simulink model "float_mch_Sample_AdaptiveThreshold"  (R2020a)
settings: Solver=VariableStepAuto  StartTime=0  StopTime=5  RelTol=1e-3
values from neighbouring files (symbols this model uses):
  fs = 30000    [float_mch_run_LocalMaxima_AdaptiveThreshold.m]    (also in float_mch_run_LocalMaxima_HardThreshold.m; float_mch_run_Sample_AdaptiveThreshold.m; float_mch_run_Sample_HardThreshold.m)
libraries: dspfdesign x2, dspswit3 x1, dspstat3 x1, simulink x1
settings Model: Creator=sbuccelli  LastModifiedBy=diflo

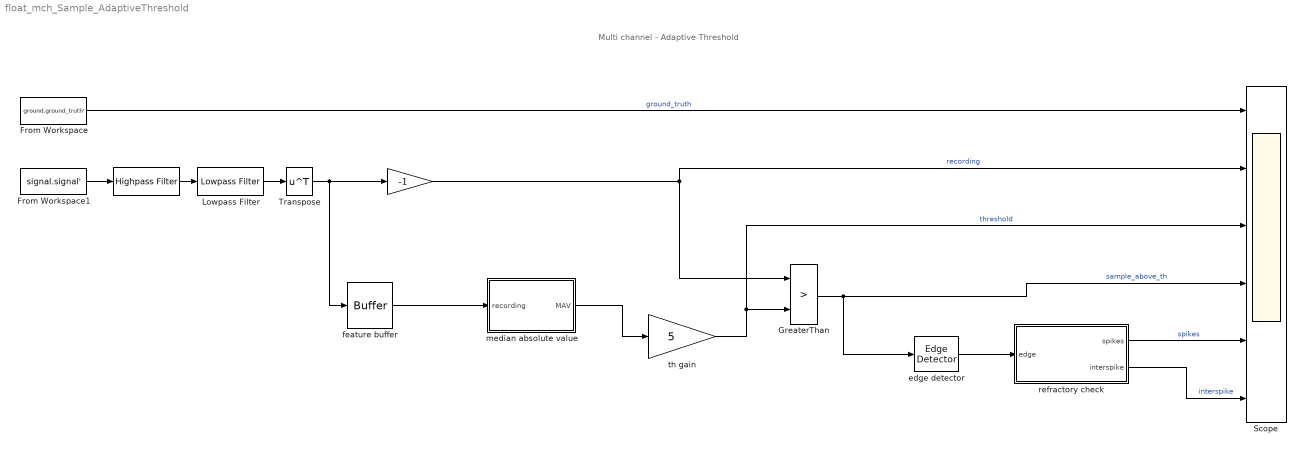
== system float_mch_Sample_AdaptiveThreshold ==
  note: Multi channel - Adaptive Threshold
  " " : Gain  Gain=-1
  "   " : dspfdesign/Highpass Filter  FilterType=IIR  DesignForMinimumOrder=on  FilterOrder=50  StopbandFrequency=1  PassbandFrequency=300  StopbandAttenuation=80  PassbandRipple=0.1  InheritSampleRate=off  SampleRate=30000  SimulateUsing=Interpreted execution  roundingMode=Floor  coeffsDataTypeStr=fixdt(1,16)
  From Workspace : FromWorkspace  VariableName=ground.ground_truth'  SampleTime=1/fs
  From Workspace1 : FromWorkspace  VariableName=signal.signal'  SampleTime=1/fs
  GreaterThan : RelationalOperator  Operator=>  OutDataTypeStr=boolean  RndMeth=Simplest
  Lowpass Filter : dspfdesign/Lowpass Filter  FilterType=IIR  DesignForMinimumOrder=on  FilterOrder=3  PassbandFrequency=3500  StopbandFrequency=8500  PassbandRipple=0.1  StopbandAttenuation=80  InheritSampleRate=off  SampleRate=30000  SimulateUsing=Interpreted execution  roundingMode=Floor  coeffsDataTypeStr=fixdt(1,16)
  Scope : Scope  NumInputPorts=6
  Transpose : Math  Operator=transpose  SaturateOnIntegerOverflow=on
  edge detector : dspswit3/Edge Detector  InputProcessing=Columns as channels (frame based)
      settings: SourceProductBaseCode=DS
  feature buffer : Buffer  N=30000  OutputFrames=off
  median absolute value : Subsystem
  refractory check : Subsystem
  th gain : Gain  Gain=5
  wires:
  From Workspace/1 -> Scope/1  "ground_truth"
  edge detector/1 -> refractory check/1("edge  ")
  refractory check/2(interspike) -> Scope/6  "interspike"
  GreaterThan/1 -> Scope/4, edge detector/1  "sample_above_th"
  th gain/1 -> GreaterThan/2, Scope/3  "threshold"
  refractory check/1(spikes) -> Scope/5  "spikes"
  From Workspace1/1 -> "   "/1
  " "/1 -> GreaterThan/1, Scope/2  "recording"
  feature buffer/1 -> median absolute value/1(recording)
  median absolute value/1(MAV) -> th gain/1
  Transpose/1 -> feature buffer/1, " "/1
  "   "/1 -> Lowpass Filter/1
  Lowpass Filter/1 -> Transpose/1

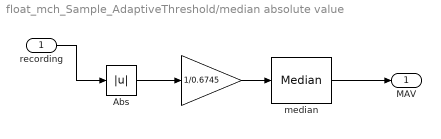
== system float_mch_Sample_AdaptiveThreshold/median absolute value ==
  recording : Inport
  "  " : Gain  Gain=1/0.6745
  Abs : Abs
  median : dspstat3/Median  sortAlg=Quick sort  directionMode=Each column  dimension=1  roundingMode=Floor  overflowMode=off  accumDataTypeStr=Inherit: Same as product output  accumLastDataTypeStr=Inherit: Same as product output  outputDataTypeStr=Inherit: Same as accumulator  outputMin=[]  outputMax=[]  outputLastDataTypeStr=Inherit: Same as accumulator
      settings: SourceProductBaseCode=DS  allowOverrides=off
  MAV : Outport
  wires:
  Abs/1 -> "  "/1
  "  "/1 -> median/1
  recording/1 -> Abs/1
  median/1 -> MAV/1

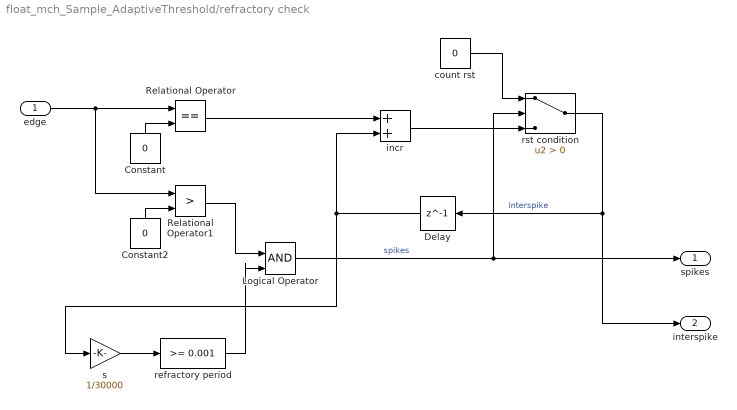
== system float_mch_Sample_AdaptiveThreshold/refractory check ==
  "edge  " : Inport
  Constant : Constant  Value=0
  Constant2 : Constant  Value=0
  Delay : Delay  DelayLength=1  InitialCondition=1
  Logical Operator : Logic  IconShape=distinctive  AllPortsSameDT=off  OutDataTypeStr=boolean
  Relational Operator : RelationalOperator  Operator===  OutDataTypeStr=boolean  RndMeth=Simplest
  Relational Operator1 : RelationalOperator  Operator=>  OutDataTypeStr=boolean  RndMeth=Simplest
  count rst : Constant  Value=0
  incr : Sum  AccumDataTypeStr=double
  refractory period : simulink/Logic and Bit Operations/Compare To Constant  relop=>=  const=0.001  OutDataTypeStr=boolean
  rst condition : Switch  Criteria=u2 > Threshold  OutDataTypeStr=double
  s : Gain  Gain=1/30000
  spikes : Outport
  interspike : Outport  Port=2
  wires:
  count rst/1 -> rst condition/1
  Constant/1 -> Relational Operator/2
  Constant2/1 -> Relational Operator1/2
  Relational Operator1/1 -> Logical Operator/1
  refractory period/1 -> Logical Operator/2
  Logical Operator/1 -> spikes/1, rst condition/2  "spikes"
  incr/1 -> rst condition/3
  rst condition/1 -> interspike/1, Delay/1  "interspike"
  Delay/1 -> s/1, incr/2
  Relational Operator/1 -> incr/1
  "edge  "/1 -> Relational Operator1/1, Relational Operator/1
  s/1 -> refractory period/1
